simulink model "radiator_simscape"  (R2016b)
settings: Solver=VariableStepAuto  StartTime=0.0  StopTime=3600*36  RelTol=1e-3
model workspace (MATLAB code in the model file):
  | radiator_simscape_data
values from neighbouring files (symbols this model uses):
  TinHeatK = 273+5    (= 278)    [radiator_simscape_data.m]
  TinIC = 5    [radiator_simscape_data.m]
libraries: fl_lib x16, nesl_utility x7, slident x1, mpclib x1
settings Model: PauseTimes=3600  NumberOfSteps=7200  Creator=Gyulai László  LastModifiedBy=Gyulai László

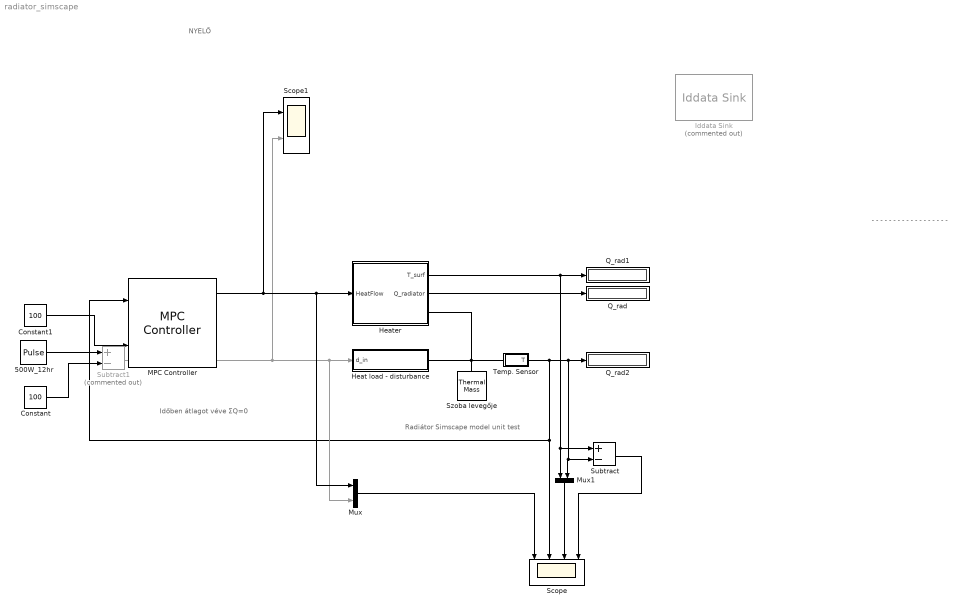
== system radiator_simscape ==
  note: Időben átlagot véve ΣQ=0
  note: - - - - - -
      |
      | - - -    - - -
      |
      | - - - - - -
  note: NYELŐ
  note: Radiátor Simscape model unit test
  500W_12hr : DiscretePulseGenerator  PulseType=Time based  Amplitude=200  Period=3600*6  PulseWidth=50
  Constant : Constant  Value=100
  Constant1 : Constant  Value=100
  Heat load - disturbance : Subsystem
  Heater : Subsystem
  Iddata Sink : slident/Iddata Sink  Commented=on  datasetname=disturb  Ts=300  isu=off  isy=off
  MPC Controller : mpclib/MPC Controller  SCDEnableBlockLinearizationSpecification=on  mpcobj=radiator_unittest_mpc_heatcontrol_Ts1  is_multiple=0  enable_value=0  return_u0=off  ref_from_ws=off  ref_signal_name=[]  ref_preview=off  md_from_ws=off  md_signal_name=[]  md_preview=off  from_project=off  project_file=MPCtask.mat  md_inport=off  mv_inport=off  cost_outport=on  return_sequence=on  return_qpstatus=off  return_state=off  state_inport=off  lims_inport=off  ywt_inport=off  is_designfromscratch=0  uwt_inport=off  duwt_inport=off  rhoeps_inport=off  uref_inport=off  n_ts=1  n_mv=1  n_md=0  n_ud=0  n_mo=1  n_uo=0  BlockDataType=double  SampleTimeInherited=off  switch_inport=off
  Mux : Mux  Inputs=2
  Mux1 : Mux  Inputs=2
  Q_rad : Display
  Q_rad1 : Display
  Q_rad2 : Display
  Scope : Scope  NumInputPorts=4
  Scope1 : Scope  NumInputPorts=2
  Subtract : Sum  Inputs=+-
  Subtract1 : Sum  Commented=on  Inputs=+-
  Szoba levegője : fl_lib/Thermal/Thermal Elements/Thermal Mass  mass=M_air kg  sp_heat=c_air J/kg/K  T_specify=on  T_priority=High  T=TinIC degC  Q_specify=off  Q_priority=None  Q=0 J/s
  Temp. Sensor : Subsystem
  wires:
  Heater/2(Q_radiator) -> Q_rad/1
  Heater/1(T_surf) -> Q_rad1/1, Mux1/1, Subtract/1
  Temp. Sensor/1(T) -> Q_rad2/1, Mux1/2, Subtract/2, Scope/2, MPC Controller/1
  Subtract1/1 -> Scope1/2, Mux/2, Heat load - disturbance/1(d_in)
  Mux1/1 -> Scope/3
  Subtract/1 -> Scope/4
  MPC Controller/1 -> Scope1/1, Heater/1(HeatFlow), Mux/1
  500W_12hr/1 -> Subtract1/1
  Constant/1 -> Subtract1/2
  Mux/1 -> Scope/1
  Constant1/1 -> MPC Controller/2
  connections:
  Szoba levegője/LConn1 -- Heater/RConn1 -- Temp. Sensor/LConn1 -- Heat load - disturbance/RConn1

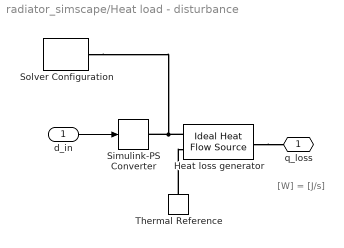
== system radiator_simscape/Heat load - disturbance ==
  note: [W] = [J/s]
  d_in : Inport
  Heat loss generator : fl_lib/Thermal/Thermal Sources/Ideal Heat Flow Source
  Simulink-PS Converter : nesl_utility/Simulink-PS Converter  PhysicalDomain=network_engine_domain  SubClassName=ps_input  LeftPortType=input  RightPortType=output  PseudoPeriodic=off  Frequencies=[]  NoiseDistribution=none  NoiseParameters=[]  Unit=1  AffineConversion=off  InputFiltering=off  SimscapeFilterOrder=1  InputFilterTimeConstant=0.001  UdotUserProvided=1
  Solver Configuration : nesl_utility/Solver Configuration  PhysicalDomain=network_engine_domain  SubClassName=solver  LeftPortType=input  RightPortType=generic  Accelerate=off  Tones=[]  Harmonics=[]  SimulateNoise=off  Profile=off  UseLocalSampling=off  EnableSwitchedLinearOptims=on  FrequencyDomain=off  UseCCode=off  RelTol=0.001  AbsTol=1e-06  MinStep=1e-09  ToWorkspace=off  RevertToSquareIcSolve=off  NumHomotopyIterations=100  PhasorMode=off  PhasorModeNumHarmonics=1  OverrideAbsTol=off  DoDC=off  ResidualTolerance=1e-9  UseLocalSolver=off  LocalSolverChoice=NE_BACKWARD_EULER_ADVANCER  LocalSolverSampleTime=.001  DoFixedCost=off  MaxNonlinIter=3  MaxModeIter=2  LinearAlgebra=Sparse  DelaysMemoryBudget=1024  AutomaticFiltering=on  FilteringTimeConstant=0.001
  Thermal Reference : fl_lib/Thermal/Thermal Elements/Thermal Reference
  q_loss : PMIOPort  Port=1  Side=Right
  wires:
  d_in/1 -> Simulink-PS Converter/1
  connections:
  Thermal Reference/LConn1 -- Heat loss generator/RConn2
  Heat loss generator/RConn1 -- Solver Configuration/RConn1 -- Simulink-PS Converter/RConn1
  Heat loss generator/LConn1 -- q_loss/RConn1

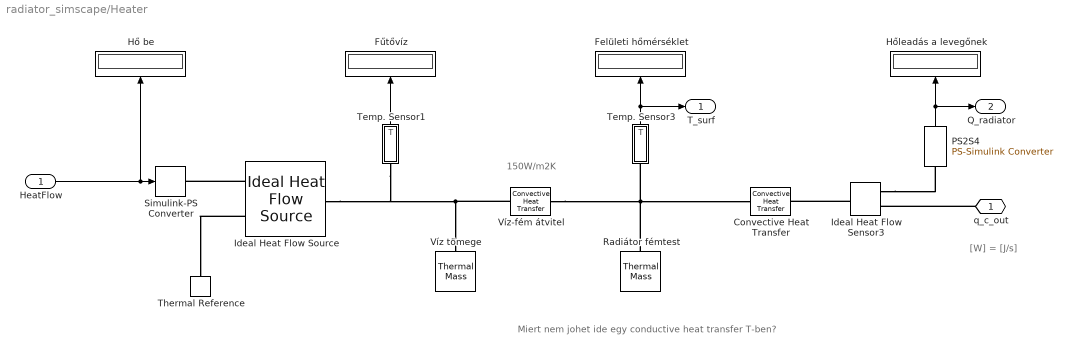
== system radiator_simscape/Heater ==
  note: Miert nem johet ide egy conductive heat transfer T-ben?
  note: [W] = [J/s]
  note: 150W/m2K
  HeatFlow : Inport
  Convective Heat Transfer : fl_lib/Thermal/Thermal Elements/Convective Heat Transfer  area=area_radiator m^2  heat_tr_coeff=h_c_radi W/(m^2 * K)  Q_specify=off  Q_priority=None  Q=0 J/s  T_specify=off  T_priority=None  T=0 K
  Felületi hőmérséklet : Display
  Fűtővíz : Display
  Hő be : Display
  Hőleadás a levegőnek : Display
  Ideal Heat Flow Sensor3 : fl_lib/Thermal/Thermal Sensors/Ideal Heat Flow Sensor
  Ideal Heat Flow Source : fl_lib/Thermal/Thermal Sources/Ideal Heat Flow Source
  PS2S4 : nesl_utility/PS-Simulink Converter  PhysicalDomain=network_engine_domain  SubClassName=ps_output  LeftPortType=input  RightPortType=output  PseudoPeriodic=off  Frequencies=[]  Unit=J/s  AffineConversion=on
  Radiátor fémtest : fl_lib/Thermal/Thermal Elements/Thermal Mass  mass=m_r kg  sp_heat=c_metal J/kg/K  T_specify=on  T_priority=High  T=TinHeatK K  Q_specify=off  Q_priority=None  Q=0 J/s
  Simulink-PS Converter : nesl_utility/Simulink-PS Converter  PhysicalDomain=network_engine_domain  SubClassName=ps_input  LeftPortType=input  RightPortType=output  PseudoPeriodic=off  Frequencies=[]  NoiseDistribution=none  NoiseParameters=[]  Unit=1  AffineConversion=off  InputFiltering=off  SimscapeFilterOrder=1  InputFilterTimeConstant=0.001  UdotUserProvided=1
  Temp. Sensor1 : Subsystem
  Temp. Sensor3 : Subsystem
  Thermal Reference : fl_lib/Thermal/Thermal Elements/Thermal Reference
  Víz tömege : fl_lib/Thermal/Thermal Elements/Thermal Mass  mass=m_w_r kg  sp_heat=c_w J/kg/K  T_specify=on  T_priority=High  T=TinHeatK K  Q_specify=off  Q_priority=None  Q=0 J/s
  Víz-fém átvitel : fl_lib/Thermal/Thermal Elements/Convective Heat Transfer  area=area_radiator m^2  heat_tr_coeff=h_w_radi W/(m^2 * K)  Q_specify=off  Q_priority=None  Q=0 J/s  T_specify=off  T_priority=None  T=0 K
  q_c_out : PMIOPort  Port=1  Side=Right
  T_surf : Outport
  Q_radiator : Outport  Port=2
  wires:
  HeatFlow/1 -> Hő be/1, Simulink-PS Converter/1
  Temp. Sensor3/1(T) -> T_surf/1, Felületi hőmérséklet/1
  Temp. Sensor1/1(T) -> Fűtővíz/1
  PS2S4/1 -> Hőleadás a levegőnek/1, Q_radiator/1
  connections:
  Ideal Heat Flow Source/RConn1 -- Simulink-PS Converter/RConn1
  Radiátor fémtest/LConn1 -- Convective Heat Transfer/LConn1 -- Temp. Sensor3/LConn1 -- Víz-fém átvitel/RConn1
  Víz-fém átvitel/LConn1 -- Ideal Heat Flow Source/LConn1 -- Temp. Sensor1/LConn1 -- Víz tömege/LConn1
  Ideal Heat Flow Source/RConn2 -- Thermal Reference/LConn1
  Ideal Heat Flow Sensor3/RConn1 -- PS2S4/LConn1
  q_c_out/RConn1 -- Ideal Heat Flow Sensor3/RConn2
  Ideal Heat Flow Sensor3/LConn1 -- Convective Heat Transfer/RConn1

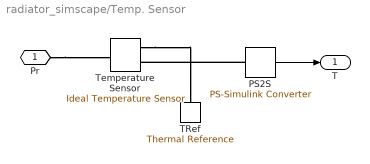
== system radiator_simscape/Temp. Sensor ==
  PS2S : nesl_utility/PS-Simulink Converter  PhysicalDomain=network_engine_domain  SubClassName=ps_output  LeftPortType=input  RightPortType=output  PseudoPeriodic=off  Frequencies=[]  Unit=degC  AffineConversion=on
  TRef : fl_lib/Thermal/Thermal Elements/Thermal Reference
  Temperature Sensor : fl_lib/Thermal/Thermal Sensors/Ideal Temperature Sensor
  Pr : PMIOPort  Port=1  Side=Left
  T : Outport
  wires:
  PS2S/1 -> T/1
  connections:
  Temperature Sensor/RConn1 -- TRef/LConn1
  PS2S/LConn1 -- Temperature Sensor/RConn2
  Pr/RConn1 -- Temperature Sensor/LConn1

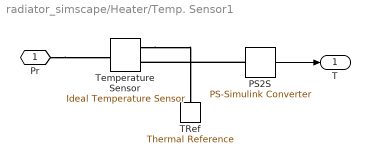
== system radiator_simscape/Heater/Temp. Sensor1 ==
  PS2S : nesl_utility/PS-Simulink Converter  PhysicalDomain=network_engine_domain  SubClassName=ps_output  LeftPortType=input  RightPortType=output  PseudoPeriodic=off  Frequencies=[]  Unit=degC  AffineConversion=on
  TRef : fl_lib/Thermal/Thermal Elements/Thermal Reference
  Temperature Sensor : fl_lib/Thermal/Thermal Sensors/Ideal Temperature Sensor
  Pr : PMIOPort  Port=1  Side=Left
  T : Outport
  wires:
  PS2S/1 -> T/1
  connections:
  Temperature Sensor/RConn1 -- TRef/LConn1
  PS2S/LConn1 -- Temperature Sensor/RConn2
  Pr/RConn1 -- Temperature Sensor/LConn1

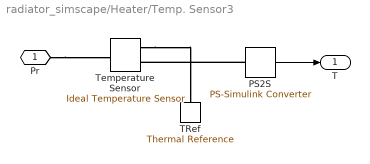
== system radiator_simscape/Heater/Temp. Sensor3 ==
  PS2S : nesl_utility/PS-Simulink Converter  PhysicalDomain=network_engine_domain  SubClassName=ps_output  LeftPortType=input  RightPortType=output  PseudoPeriodic=off  Frequencies=[]  Unit=degC  AffineConversion=on
  TRef : fl_lib/Thermal/Thermal Elements/Thermal Reference
  Temperature Sensor : fl_lib/Thermal/Thermal Sensors/Ideal Temperature Sensor
  Pr : PMIOPort  Port=1  Side=Left
  T : Outport
  wires:
  PS2S/1 -> T/1
  connections:
  Temperature Sensor/RConn1 -- TRef/LConn1
  PS2S/LConn1 -- Temperature Sensor/RConn2
  Pr/RConn1 -- Temperature Sensor/LConn1
